simulink model "physbe"  (Simulink 9.0)
settings: Solver=ode45  StartTime=0.0  StopTime=20  FixedStep=1/1000  MaxStep=1/10  RelTol=1e-3  AbsTol=1e-6
PreLoadFcn:
  | pctrl2
values from neighbouring files (symbols this model uses):
  A = [  0.0   0.0   0.0  0.0  3.67   1.4   6.0   7.0  0.0  0.0 ]'*1000    [pctrl2.m]    (also in physbe_settings.mat = [0 0 0 0 3670 1400 6000 7000 0 0])
  C = [   75  5.33 75.00 1.01  4.25  1.21  34.0  11.1  250 32.5 ]'    [pctrl2.m]    (also in physbe_settings.mat = [75 7.519 80 1.25 4.25 1.21 34 11.1 250 30.3 2.57 5.33 ... ()
  Cl = [ 0.0000 0.04 0.08 0.12 0.16 0.20 0.24 0.28 0.32 0.36 0.4000 1.0000 ... (first row only)    [pctrl2.m]    (also in physbe_settings.mat = [0 0.00264 0.016 0.24 0.032 0.4 0.048 0.5 0.064 0.56 0.08 0.)
  Cr = [ 0.0000 0.04 0.08 0.12 0.16 0.20 0.24 0.28 0.32 0.36 0.4000 1.0000 ... (first row only)    [pctrl2.m]    (also in physbe_settings.mat = [0 0.00132 0.016 0.02 0.032 0.04 0.048 0.06 0.064 0.068 0.08)
  fd = fe    [pctrl2.m]    (also in physbe_settings.mat = [0 0 0 0 0 0 0 0 0 0])
  fe = [  0.0   0.0   0.0  0.0   0.0   0.0   0.0   0.0  0.0  0.0 ]'    [pctrl2.m]    (also in physbe_settings.mat = [0 0 0 0 0 0 0 0 0 0])
  h0 = [  0.0   0.0   0.0  0.0   0.0   0.0   0.0   0.0  0.0  0.0 ]'    [pctrl2.m]    (also in physbe_settings.mat = [0 0 0 0 0 0 0 0 0 0 0 0 ... (20 elements, 10x2)])
  K = 1    [pctrl2.m]    (also in physbe_settings.mat)
  Ri = [  3.0 187.5  27.5    0  5150  2580   670  2580  0.0  0.0 ]'*0.001    [pctrl2.m]    (also in physbe_settings.mat = [0.0128 0.1429 0.0588 0 5.15 2.58 0.67 2.58 0 0])
  Ro = [ 3e-3   0.0  6e-3    0    10     5  1.42     5  0.0  0.0 ]'    [pctrl2.m]    (also in physbe_settings.mat = [0.0111 0 0.0125 0 10 5 1.42 5 0 0])
  ta = 300    [pctrl2.m]    (also in physbe_settings.mat)
  V0 = [  150   120   150  100   280  80.0  2250   730  500  240 ]'    [pctrl2.m]    (also in physbe_settings.mat = [150 120 150 100 280 80 2250 730 500 240 2.57 120 ... (20 el)
  W = [  0.6   1.0   0.6  0.0  7.00   4.5  53.0  18.5  0.0  0.0 ]'*1000    [pctrl2.m]    (also in physbe_settings.mat = [600 1000 600 0 7000 4500 53000 18500 0 0])
libraries: simulink x2
CloseFcn:
  | close(findobj(allchild(0),'flat','name','PHYSBE Control Center'))
settings Model: Creator=anast  LastModifiedBy=anast  ExtModeTrigMode=oneshot  ExtModeArmWhenConnect=off
settings DataIOCC: Decimation=10  LimitDataPoints=on  SignalLoggingSaveFormat=ModelDataLogs
settings OptimizationCC: BlockReduction=off  BooleanDataType=off  LifeSpan=auto
settings DebuggingCC: ConsistencyChecking=warning  SaveWithParameterizedLinksMsg=none  SignalResolutionControl=TryResolveAllWithWarning  MultiTaskDSMMsg=warning  MultiTaskCondExecSysMsg=none  SFUnexpectedBacktrackingDiag=error  SFNoUnconditionalDefaultTransitionDiag=error  SFExecutionAtInitializationDiag=warning
settings HardwareCC: ProdBitPerPointer=64  ProdBitPerSizeT=64  ProdBitPerPtrDiffT=64  ProdLargestAtomicFloat=Float  ProdIntDivRoundTo=Zero  ProdEndianess=LittleEndian  ProdWordSize=64  ProdHWDeviceType=Intel->x86-64 (Windows64)  TargetUnknown=on
settings CodeAppCC: StateflowObjectComments=off
settings GRTTargetCC: CombineOutputUpdateFcns=off  GRTInterface=on
settings ConfigComp: CovMetricSettings=dwe  CovHtmlReporting=off  CovSaveCumulativeToWorkspaceVar=off  CovSaveSingleToWorkspaceVar=off  CovExternalEMLEnable=on

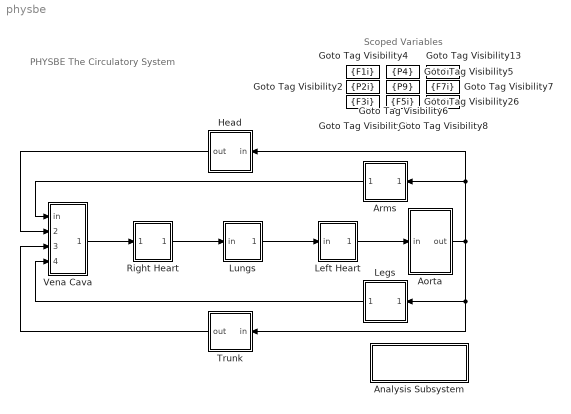
== system physbe ==
  note: Scoped Variables
  note: PHYSBE
      |  The Circulatory System
  Analysis Subsystem : Subsystem
      mask Display: disp('Analysis\nSubsystem')
  Aorta : Subsystem
      mask Display: disp('AORTA')
  Arms : Subsystem
      mask Display: disp('ARMS')
  Goto Tag Visibility13 : GotoTagVisibility  GotoTag=F6i
  Goto Tag Visibility2 : GotoTagVisibility  GotoTag=P2i
  Goto Tag Visibility26 : GotoTagVisibility  GotoTag=F5i
  Goto Tag Visibility3 : GotoTagVisibility  GotoTag=F3i
  Goto Tag Visibility4 : GotoTagVisibility  GotoTag=F1i
  Goto Tag Visibility5 : GotoTagVisibility  GotoTag=P4
  Goto Tag Visibility6 : GotoTagVisibility  GotoTag=P9
  Goto Tag Visibility7 : GotoTagVisibility  GotoTag=F7i
  Goto Tag Visibility8 : GotoTagVisibility  GotoTag=F8i
  Head : Subsystem
      mask Display: disp('HEAD')
  Left Heart : Subsystem
      mask Display: disp(' LEFT\n HEART')
  Legs : Subsystem
      mask Display: disp('LEGS')
  Lungs : Subsystem
      mask Display: disp('LUNGS')
  Right Heart : Subsystem
      mask Display: disp(' RIGHT\n HEART')
  Trunk : Subsystem
      mask Display: disp('TRUNK')
  Vena Cava : Subsystem
      mask Display: disp('VENA\nCAVA')
  wires:
  Arms/1(out1) -> Vena Cava/1(in)
  Head/1(out) -> Vena Cava/2(in1)
  Aorta/1(out) -> Legs/1(in1), Trunk/1(in), Arms/1(in1), Head/1(in)
  Lungs/1(out) -> Left Heart/1(in)
  Right Heart/1(out1) -> Lungs/1(in)
  Vena Cava/1(out) -> Right Heart/1(in1)
  Left Heart/1(out) -> Aorta/1(in)
  Legs/1(out1) -> Vena Cava/4(in3)
  Trunk/1(out) -> Vena Cava/3(in2)

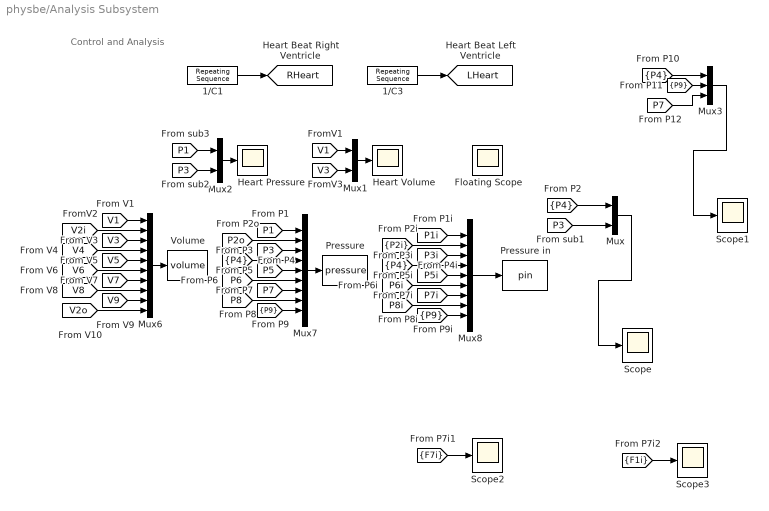
== system physbe/Analysis Subsystem ==
  note: Control
      | and
      |  Analysis
  1/C1 : simulink/Sources/Repeating Sequence  rep_seq_t=Cr(1,:)  rep_seq_y=Cr(2,:)
  1/C3 : simulink/Sources/Repeating Sequence  rep_seq_t=Cl(1,:)  rep_seq_y=Cl(2,:)
  Floating Scope : Scope
      settings: Floating=on
  Heart Pressure : Scope
  Heart Volume : Scope
  Mux : Mux  Inputs=2
  Mux1 : Mux  Inputs=2
  Mux2 : Mux  Inputs=2
  Mux3 : Mux  Inputs=3
  Mux6 : Mux  Inputs=10
  Mux7 : Mux  Inputs=9
  Mux8 : Mux  Inputs=9
  Pressure : ToWorkspace  VariableName=pressure  SampleTime=-1
      settings: Decimation=10
  Pressure in : ToWorkspace  VariableName=pin  SampleTime=-1
      settings: Decimation=10
  Scope{,1..3} (4 alike) : Scope
  Volume : ToWorkspace  VariableName=volume  SampleTime=-1
      settings: Decimation=10
  tag scope: LHeart=global, RHeart=global
  wires:
  Mux8/1 -> Pressure in/1
  [P7i] -> Mux8/7
  [P5i] -> Mux8/5
  [P3i] -> Mux8/3
  [P1i] -> Mux8/1
  [P9] -> Mux8/9
  [P7] -> Mux7/7
  [P3] -> Mux7/3
  [P5] -> Mux7/5
  [P9] -> Mux7/9
  Mux7/1 -> Pressure/1
  [P1] -> Mux7/1
  [V2o] -> Mux6/10
  [V2i] -> Mux6/2
  [V6] -> Mux6/6
  [V4] -> Mux6/4
  [V5] -> Mux6/5
  [V3] -> Mux6/3
  [V7] -> Mux6/7
  [V8] -> Mux6/8
  Mux6/1 -> Volume/1
  [V9] -> Mux6/9
  [V1] -> Mux6/1
  [P2o] -> Mux7/2
  [P6] -> Mux7/6
  [P8] -> Mux7/8
  [P4] -> Mux7/4
  [P8i] -> Mux8/8
  [P6i] -> Mux8/6
  [P4] -> Mux8/4
  [P2i] -> Mux8/2
  [P1] -> Mux2/1
  [V1] -> Mux1/1
  Mux1/1 -> Heart Volume/1
  [P3] -> Mux2/2
  Mux2/1 -> Heart Pressure/1
  [V3] -> Mux1/2
  1/C3/1 -> [LHeart]
  1/C1/1 -> [RHeart]
  [P3] -> Mux/2
  Mux/1 -> Scope/1
  [P4] -> Mux/1
  Mux3/1 -> Scope1/1
  [P4] -> Mux3/1
  [P9] -> Mux3/2
  [P7] -> Mux3/3
  [F7i] -> Scope2/1
  [F1i] -> Scope3/1

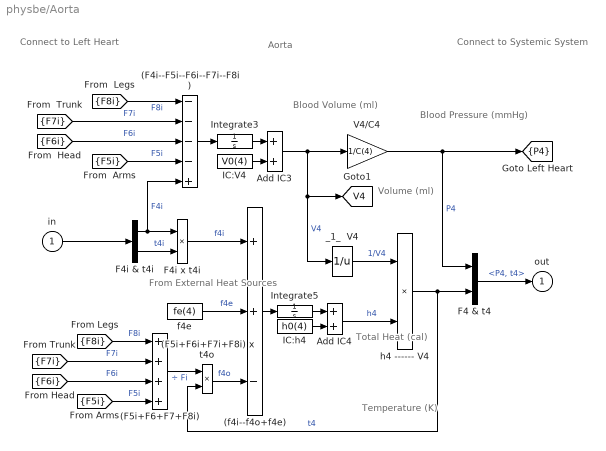
== system physbe/Aorta ==
  note: Temperature
      | (K)
  note: Volume
      | (ml)
  note: Connect to
      | Left Heart
  note: Connect to
      | Systemic System
  note: From External
      | Heat Sources
  note: Blood
      | Pressure
      | (mmHg)
  note: Total
      | Heat
      | (cal)
  note: Blood
      |  Volume
      | (ml)
  note: Aorta
  in : Inport
  (F4i--F5i--F6i--F7i--F8i) : Sum  Inputs=----+  SaturateOnIntegerOverflow=on  InputSameDT=on  OutDataTypeStr=Inherit: Same as first input
  (F5i+F6+F7+F8i) : Sum  Inputs=++++  SaturateOnIntegerOverflow=on  InputSameDT=on  OutDataTypeStr=Inherit: Same as first input
  (F5i+F6i+F7i+F8i) x t4o : Product  SaturateOnIntegerOverflow=on  RndMeth=Zero  InputSameDT=on  OutDataTypeStr=Inherit: Same as first input
  (f4i--f4o+f4e) : Sum  Inputs=++-  SaturateOnIntegerOverflow=on  InputSameDT=on  OutDataTypeStr=Inherit: Same as first input
  Add IC3 : Sum  SaturateOnIntegerOverflow=on  InputSameDT=on  OutDataTypeStr=Inherit: Same as first input
  Add IC4 : Sum  SaturateOnIntegerOverflow=on  InputSameDT=on  OutDataTypeStr=Inherit: Same as first input
  F4 & t4 : Mux  Inputs=2
  F4i & t4i : Demux  Outputs=2
  F4i x t4i : Product  SaturateOnIntegerOverflow=on  RndMeth=Zero  InputSameDT=on  OutDataTypeStr=Inherit: Same as first input
  IC:V4 : Constant  Value=V0(4)
  IC:h4 : Constant  Value=h0(4)
  Integrate3 : Integrator
  Integrate5 : Integrator
  V4/C4 : Gain  Gain=1/C(4)  SaturateOnIntegerOverflow=on  OutDataTypeStr=Inherit: Same as input  ParamDataTypeStr=Inherit: Same as input
  _1_  V4 : Math  Operator=reciprocal  SaturateOnIntegerOverflow=on
  f4e : Constant  Value=fe(4)
  h4 ------ V4 : Product  SaturateOnIntegerOverflow=on  RndMeth=Zero  InputSameDT=on  OutDataTypeStr=Inherit: Same as first input
  out : Outport
  tag scope: P4=scoped, V4=global
  wires:
  Integrate5/1 -> Add IC4/1
  IC:h4/1 -> Add IC4/2
  Integrate3/1 -> Add IC3/1
  IC:V4/1 -> Add IC3/2
  F4 & t4/1 -> out/1  "<P4, t4>"
  [F7i] -> (F4i--F5i--F6i--F7i--F8i)/2  "F7i"
  [F6i] -> (F4i--F5i--F6i--F7i--F8i)/3  "F6i"
  in/1 -> F4i & t4i/1
  [F7i] -> (F5i+F6+F7+F8i)/2  "F7i"
  [F6i] -> (F5i+F6+F7+F8i)/3  "F6i"
  [F8i] -> (F5i+F6+F7+F8i)/1  "F8i"
  [F5i] -> (F5i+F6+F7+F8i)/4  "F5i"
  (F5i+F6+F7+F8i)/1 -> (F5i+F6i+F7i+F8i) x t4o/1  "÷ Fi"
  F4i x t4i/1 -> (f4i--f4o+f4e)/1  "f4i"
  F4i & t4i/1 -> F4i x t4i/1, (F4i--F5i--F6i--F7i--F8i)/5  "F4i"
  F4i & t4i/2 -> F4i x t4i/2  "t4i"
  f4e/1 -> (f4i--f4o+f4e)/2  "f4e"
  [F8i] -> (F4i--F5i--F6i--F7i--F8i)/1  "F8i"
  [F5i] -> (F4i--F5i--F6i--F7i--F8i)/4  "F5i"
  V4/C4/1 -> [P4], F4 & t4/1  "P4"
  Add IC3/1 -> V4/C4/1, _1_  V4/1, [V4]  "V4"
  Add IC4/1 -> h4 ------ V4/2  "h4"
  _1_  V4/1 -> h4 ------ V4/1  "1/V4"
  h4 ------ V4/1 -> (F5i+F6i+F7i+F8i) x t4o/2, F4 & t4/2  "t4"
  (f4i--f4o+f4e)/1 -> Integrate5/1
  (F5i+F6i+F7i+F8i) x t4o/1 -> (f4i--f4o+f4e)/3  "f4o"
  (F4i--F5i--F6i--F7i--F8i)/1 -> Integrate3/1

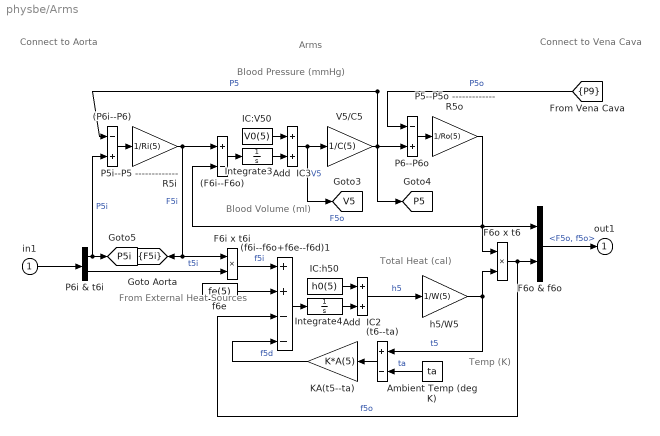
== system physbe/Arms ==
  note: From External
      | Heat Sources
  note: Blood Volume
      | (ml)
  note: Blood Pressure (mmHg)
  note: Total
      | Heat
      |  (cal)
  note: Temp
      | (K)
  note: Connect to
      | Vena Cava
  note: Arms
  note: Connect to
      | Aorta
  in1 : Inport
  (F6i--F6o) : Sum  Inputs=+-  SaturateOnIntegerOverflow=on  InputSameDT=on  OutDataTypeStr=Inherit: Same as first input
  (P6i--P6) : Sum  Inputs=-+  SaturateOnIntegerOverflow=on  InputSameDT=on  OutDataTypeStr=Inherit: Same as first input
  (f6i--f6o+f6e--f6d)1 : Sum  Inputs=++--  SaturateOnIntegerOverflow=on  InputSameDT=on  OutDataTypeStr=Inherit: Same as first input
  (t6--ta) : Sum  Inputs=+-  SaturateOnIntegerOverflow=on  InputSameDT=on  OutDataTypeStr=Inherit: Same as first input
  Add  IC2 : Sum  SaturateOnIntegerOverflow=on  InputSameDT=on  OutDataTypeStr=Inherit: Same as first input
  Add  IC3 : Sum  SaturateOnIntegerOverflow=on  InputSameDT=on  OutDataTypeStr=Inherit: Same as first input
  Ambient Temp (deg K) : Constant  Value=ta
  F6i x t6i : Product  SaturateOnIntegerOverflow=on  RndMeth=Zero  InputSameDT=on  OutDataTypeStr=Inherit: Same as first input
  F6o & f6o : Mux  Inputs=2
  F6o x t6 : Product  SaturateOnIntegerOverflow=on  RndMeth=Zero  InputSameDT=on  OutDataTypeStr=Inherit: Same as first input
  IC:V50 : Constant  Value=V0(5)
  IC:h50 : Constant  Value=h0(5)
  Integrate3 : Integrator
  Integrate4 : Integrator
  KA(t5--ta) : Gain  Gain=K*A(5)  SaturateOnIntegerOverflow=on  OutDataTypeStr=Inherit: Same as input  ParamDataTypeStr=Inherit: Same as input
  P5--P5o ------------- R5o : Gain  Gain=1/Ro(5)  SaturateOnIntegerOverflow=on  OutDataTypeStr=Inherit: Same as input  ParamDataTypeStr=Inherit: Same as input
  P5i--P5 ------------- R5i : Gain  Gain=1/Ri(5)  SaturateOnIntegerOverflow=on  OutDataTypeStr=Inherit: Same as input  ParamDataTypeStr=Inherit: Same as input
  P6--P6o : Sum  Inputs=-+  SaturateOnIntegerOverflow=on  InputSameDT=on  OutDataTypeStr=Inherit: Same as first input
  P6i & t6i : Demux  Outputs=2
  V5/C5 : Gain  Gain=1/C(5)  SaturateOnIntegerOverflow=on  OutDataTypeStr=Inherit: Same as input  ParamDataTypeStr=Inherit: Same as input
  f6e : Constant  Value=fe(5)
  h5/W5 : Gain  Gain=1/W(5)  SaturateOnIntegerOverflow=on  OutDataTypeStr=Inherit: Same as input  ParamDataTypeStr=Inherit: Same as input
  out1 : Outport
  tag scope: F5i=scoped, P5=global, P5i=global, V5=global
  wires:
  P6i & t6i/1 -> [P5i], (P6i--P6)/2  "P5i"
  h5/W5/1 -> (t6--ta)/1, F6o x t6/2  "t5"
  Ambient Temp (deg K)/1 -> (t6--ta)/2  "ta"
  (t6--ta)/1 -> KA(t5--ta)/1
  KA(t5--ta)/1 -> (f6i--f6o+f6e--f6d)1/4  "f5d"
  P5--P5o ------------- R5o/1 -> F6o x t6/1, F6o & f6o/1, (F6i--F6o)/2  "F5o"
  P6--P6o/1 -> P5--P5o ------------- R5o/1
  [P9] -> P6--P6o/1  "P5o"
  V5/C5/1 -> P6--P6o/2, (P6i--P6)/1, [P5]  "P5"
  Add  IC3/1 -> V5/C5/1, [V5]  "V5"
  Integrate3/1 -> Add  IC3/2
  IC:V50/1 -> Add  IC3/1
  F6o x t6/1 -> F6o & f6o/2, (f6i--f6o+f6e--f6d)1/3  "f5o"
  F6o & f6o/1 -> out1/1  "<F5o, f5o>"
  IC:h50/1 -> Add  IC2/1
  Integrate4/1 -> Add  IC2/2
  Add  IC2/1 -> h5/W5/1  "h5"
  f6e/1 -> (f6i--f6o+f6e--f6d)1/2
  F6i x t6i/1 -> (f6i--f6o+f6e--f6d)1/1  "f5i"
  (f6i--f6o+f6e--f6d)1/1 -> Integrate4/1
  P6i & t6i/2 -> F6i x t6i/2  "t5i"
  (P6i--P6)/1 -> P5i--P5 ------------- R5i/1
  P5i--P5 ------------- R5i/1 -> (F6i--F6o)/1, [F5i], F6i x t6i/1  "F5i"
  (F6i--F6o)/1 -> Integrate3/1
  in1/1 -> P6i & t6i/1

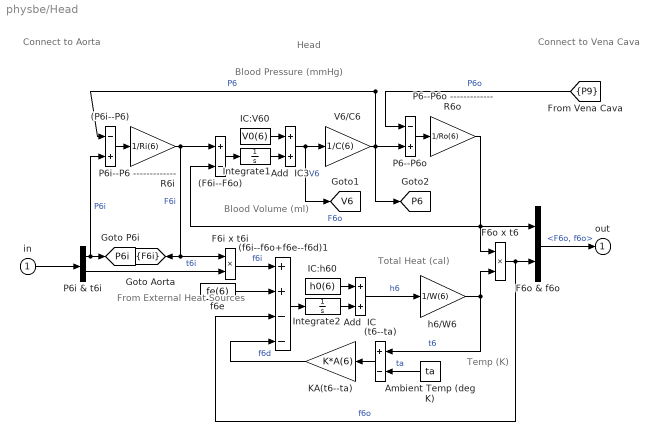
== system physbe/Head ==
  note: Connect to
      | Vena Cava
  note: From External
      | Heat Sources
  note: Head
  note: Blood Volume
      | (ml)
  note: Blood Pressure (mmHg)
  note: Total
      | Heat
      |  (cal)
  note: Temp
      | (K)
  note: Connect to
      | Aorta
  in : Inport
  (F6i--F6o) : Sum  Inputs=+-  SaturateOnIntegerOverflow=on  InputSameDT=on  OutDataTypeStr=Inherit: Same as first input
  (P6i--P6) : Sum  Inputs=-+  SaturateOnIntegerOverflow=on  InputSameDT=on  OutDataTypeStr=Inherit: Same as first input
  (f6i--f6o+f6e--f6d)1 : Sum  Inputs=++--  SaturateOnIntegerOverflow=on  InputSameDT=on  OutDataTypeStr=Inherit: Same as first input
  (t6--ta) : Sum  Inputs=+-  SaturateOnIntegerOverflow=on  InputSameDT=on  OutDataTypeStr=Inherit: Same as first input
  Add  IC : Sum  SaturateOnIntegerOverflow=on  InputSameDT=on  OutDataTypeStr=Inherit: Same as first input
  Add  IC3 : Sum  SaturateOnIntegerOverflow=on  InputSameDT=on  OutDataTypeStr=Inherit: Same as first input
  Ambient Temp (deg K) : Constant  Value=ta
  F6i x t6i : Product  SaturateOnIntegerOverflow=on  RndMeth=Zero  InputSameDT=on  OutDataTypeStr=Inherit: Same as first input
  F6o & f6o : Mux  Inputs=2
  F6o x t6 : Product  SaturateOnIntegerOverflow=on  RndMeth=Zero  InputSameDT=on  OutDataTypeStr=Inherit: Same as first input
  IC:V60 : Constant  Value=V0(6)
  IC:h60 : Constant  Value=h0(6)
  Integrate1 : Integrator
  Integrate2 : Integrator
  KA(t6--ta) : Gain  Gain=K*A(6)  SaturateOnIntegerOverflow=on  OutDataTypeStr=Inherit: Same as input  ParamDataTypeStr=Inherit: Same as input
  P6--P6o : Sum  Inputs=-+  SaturateOnIntegerOverflow=on  InputSameDT=on  OutDataTypeStr=Inherit: Same as first input
  P6--P6o ------------- R6o : Gain  Gain=1/Ro(6)  SaturateOnIntegerOverflow=on  OutDataTypeStr=Inherit: Same as input  ParamDataTypeStr=Inherit: Same as input
  P6i & t6i : Demux  Outputs=2
  P6i--P6 ------------- R6i : Gain  Gain=1/Ri(6)  SaturateOnIntegerOverflow=on  OutDataTypeStr=Inherit: Same as input  ParamDataTypeStr=Inherit: Same as input
  V6/C6 : Gain  Gain=1/C(6)  SaturateOnIntegerOverflow=on  OutDataTypeStr=Inherit: Same as input  ParamDataTypeStr=Inherit: Same as input
  f6e : Constant  Value=fe(6)
  h6/W6 : Gain  Gain=1/W(6)  SaturateOnIntegerOverflow=on  OutDataTypeStr=Inherit: Same as input  ParamDataTypeStr=Inherit: Same as input
  out : Outport
  tag scope: F6i=scoped, P6=global, P6i=global, V6=global
  wires:
  P6i & t6i/1 -> [P6i], (P6i--P6)/2  "P6i"
  h6/W6/1 -> (t6--ta)/1, F6o x t6/2  "t6"
  Ambient Temp (deg K)/1 -> (t6--ta)/2  "ta"
  (t6--ta)/1 -> KA(t6--ta)/1
  KA(t6--ta)/1 -> (f6i--f6o+f6e--f6d)1/4  "f6d"
  P6--P6o ------------- R6o/1 -> F6o x t6/1, F6o & f6o/1, (F6i--F6o)/2  "F6o"
  P6--P6o/1 -> P6--P6o ------------- R6o/1
  [P9] -> P6--P6o/1  "P6o"
  V6/C6/1 -> P6--P6o/2, (P6i--P6)/1, [P6]  "P6"
  Add  IC3/1 -> V6/C6/1, [V6]  "V6"
  F6o x t6/1 -> F6o & f6o/2, (f6i--f6o+f6e--f6d)1/3  "f6o"
  F6o & f6o/1 -> out/1  "<F6o, f6o>"
  IC:h60/1 -> Add  IC/1
  Integrate2/1 -> Add  IC/2
  Add  IC/1 -> h6/W6/1  "h6"
  f6e/1 -> (f6i--f6o+f6e--f6d)1/2
  F6i x t6i/1 -> (f6i--f6o+f6e--f6d)1/1  "f6i"
  (f6i--f6o+f6e--f6d)1/1 -> Integrate2/1
  P6i & t6i/2 -> F6i x t6i/2  "t6i"
  in/1 -> P6i & t6i/1
  (P6i--P6)/1 -> P6i--P6 ------------- R6i/1
  P6i--P6 ------------- R6i/1 -> (F6i--F6o)/1, [F6i], F6i x t6i/1  "F6i"
  Integrate1/1 -> Add  IC3/2
  (F6i--F6o)/1 -> Integrate1/1
  IC:V60/1 -> Add  IC3/1

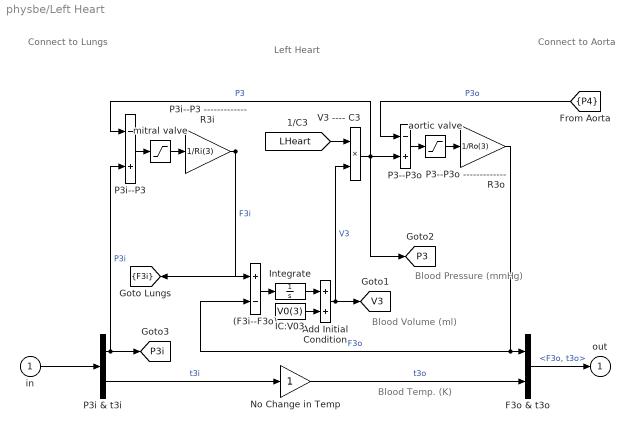
== system physbe/Left Heart ==
  note: Left Heart
  note: Connect to
      | Lungs
  note: Blood Volume (ml)
  note: Blood Pressure
      | (mmHg)
  note: Connect to
      | Aorta
  note: Blood Temp. (K)
  in : Inport
  (F3i--F3o) : Sum  Inputs=+-  SaturateOnIntegerOverflow=on  InputSameDT=on  OutDataTypeStr=Inherit: Same as first input
  Add Initial Condition : Sum  SaturateOnIntegerOverflow=on  InputSameDT=on  OutDataTypeStr=Inherit: Same as first input
  F3o & t3o : Mux  Inputs=2
  IC:V03 : Constant  Value=V0(3)
  Integrate : Integrator
  No Change in Temp : Gain  SaturateOnIntegerOverflow=on  OutDataTypeStr=Inherit: Same as input  ParamDataTypeStr=Inherit: Same as input
  P3--P3o : Sum  Inputs=-+  SaturateOnIntegerOverflow=on  InputSameDT=on  OutDataTypeStr=Inherit: Same as first input
  P3--P3o ------------- R3o : Gain  Gain=1/Ro(3)  SaturateOnIntegerOverflow=on  OutDataTypeStr=Inherit: Same as input  ParamDataTypeStr=Inherit: Same as input
  P3i & t3i : Demux  Outputs=2
  P3i--P3 : Sum  Inputs=-+  SaturateOnIntegerOverflow=on  InputSameDT=on  OutDataTypeStr=Inherit: Same as first input
  P3i--P3 ------------- R3i : Gain  Gain=1/Ri(3)  SaturateOnIntegerOverflow=on  OutDataTypeStr=Inherit: Same as input  ParamDataTypeStr=Inherit: Same as input
  V3 ---- C3 : Product  SaturateOnIntegerOverflow=on  RndMeth=Zero  InputSameDT=on  OutDataTypeStr=Inherit: Same as first input
  aortic valve : Saturate  UpperLimit=inf  LowerLimit=0
  mitral valve : Saturate  UpperLimit=inf  LowerLimit=0
  out : Outport
  tag scope: F3i=scoped, P3=global, P3i=global, V3=global
  wires:
  P3i & t3i/1 -> [P3i], P3i--P3/2  "P3i"
  P3i--P3 ------------- R3i/1 -> [F3i], (F3i--F3o)/1  "F3i"
  P3i--P3/1 -> mitral valve/1
  mitral valve/1 -> P3i--P3 ------------- R3i/1
  in/1 -> P3i & t3i/1
  Add Initial Condition/1 -> [V3], V3 ---- C3/2  "V3"
  P3i & t3i/2 -> No Change in Temp/1  "t3i"
  (F3i--F3o)/1 -> Integrate/1
  Integrate/1 -> Add Initial Condition/1
  IC:V03/1 -> Add Initial Condition/2
  [LHeart] -> V3 ---- C3/1
  P3--P3o/1 -> aortic valve/1
  aortic valve/1 -> P3--P3o ------------- R3o/1
  V3 ---- C3/1 -> P3i--P3/1, [P3], P3--P3o/2  "P3"
  No Change in Temp/1 -> F3o & t3o/2  "t3o"
  F3o & t3o/1 -> out/1  "<F3o, t3o>"
  P3--P3o ------------- R3o/1 -> F3o & t3o/1, (F3i--F3o)/2  "F3o"
  [P4] -> P3--P3o/1  "P3o"

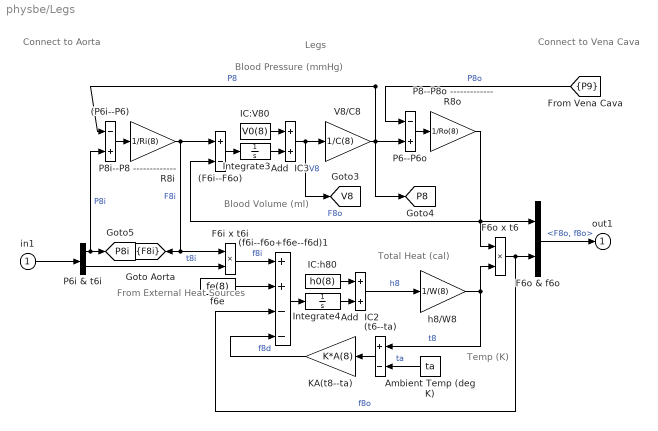
== system physbe/Legs ==
  note: From External
      | Heat Sources
  note: Blood Volume
      | (ml)
  note: Blood Pressure (mmHg)
  note: Total
      | Heat
      |  (cal)
  note: Temp
      | (K)
  note: Connect to
      | Vena Cava
  note: Legs
  note: Connect to
      | Aorta
  in1 : Inport
  (F6i--F6o) : Sum  Inputs=+-  SaturateOnIntegerOverflow=on  InputSameDT=on  OutDataTypeStr=Inherit: Same as first input
  (P6i--P6) : Sum  Inputs=-+  SaturateOnIntegerOverflow=on  InputSameDT=on  OutDataTypeStr=Inherit: Same as first input
  (f6i--f6o+f6e--f6d)1 : Sum  Inputs=++--  SaturateOnIntegerOverflow=on  InputSameDT=on  OutDataTypeStr=Inherit: Same as first input
  (t6--ta) : Sum  Inputs=+-  SaturateOnIntegerOverflow=on  InputSameDT=on  OutDataTypeStr=Inherit: Same as first input
  Add  IC2 : Sum  SaturateOnIntegerOverflow=on  InputSameDT=on  OutDataTypeStr=Inherit: Same as first input
  Add  IC3 : Sum  SaturateOnIntegerOverflow=on  InputSameDT=on  OutDataTypeStr=Inherit: Same as first input
  Ambient Temp (deg K) : Constant  Value=ta
  F6i x t6i : Product  SaturateOnIntegerOverflow=on  RndMeth=Zero  InputSameDT=on  OutDataTypeStr=Inherit: Same as first input
  F6o & f6o : Mux  Inputs=2
  F6o x t6 : Product  SaturateOnIntegerOverflow=on  RndMeth=Zero  InputSameDT=on  OutDataTypeStr=Inherit: Same as first input
  IC:V80 : Constant  Value=V0(8)
  IC:h80 : Constant  Value=h0(8)
  Integrate3 : Integrator
  Integrate4 : Integrator
  KA(t8--ta) : Gain  Gain=K*A(8)  SaturateOnIntegerOverflow=on  OutDataTypeStr=Inherit: Same as input  ParamDataTypeStr=Inherit: Same as input
  P6--P6o : Sum  Inputs=-+  SaturateOnIntegerOverflow=on  InputSameDT=on  OutDataTypeStr=Inherit: Same as first input
  P6i & t6i : Demux  Outputs=2
  P8--P8o ------------- R8o : Gain  Gain=1/Ro(8)  SaturateOnIntegerOverflow=on  OutDataTypeStr=Inherit: Same as input  ParamDataTypeStr=Inherit: Same as input
  P8i--P8 ------------- R8i : Gain  Gain=1/Ri(8)  SaturateOnIntegerOverflow=on  OutDataTypeStr=Inherit: Same as input  ParamDataTypeStr=Inherit: Same as input
  V8/C8 : Gain  Gain=1/C(8)  SaturateOnIntegerOverflow=on  OutDataTypeStr=Inherit: Same as input  ParamDataTypeStr=Inherit: Same as input
  f6e : Constant  Value=fe(8)
  h8/W8 : Gain  Gain=1/W(8)  SaturateOnIntegerOverflow=on  OutDataTypeStr=Inherit: Same as input  ParamDataTypeStr=Inherit: Same as input
  out1 : Outport
  tag scope: F8i=scoped, P8=global, P8i=global, V8=global
  wires:
  P6i & t6i/1 -> [P8i], (P6i--P6)/2  "P8i"
  h8/W8/1 -> (t6--ta)/1, F6o x t6/2  "t8"
  Ambient Temp (deg K)/1 -> (t6--ta)/2  "ta"
  (t6--ta)/1 -> KA(t8--ta)/1
  KA(t8--ta)/1 -> (f6i--f6o+f6e--f6d)1/4  "f8d"
  P8--P8o ------------- R8o/1 -> F6o x t6/1, F6o & f6o/1, (F6i--F6o)/2  "F8o"
  P6--P6o/1 -> P8--P8o ------------- R8o/1
  [P9] -> P6--P6o/1  "P8o"
  V8/C8/1 -> P6--P6o/2, (P6i--P6)/1, [P8]  "P8"
  Add  IC3/1 -> V8/C8/1, [V8]  "V8"
  Integrate3/1 -> Add  IC3/2
  IC:V80/1 -> Add  IC3/1
  F6o x t6/1 -> F6o & f6o/2, (f6i--f6o+f6e--f6d)1/3  "f8o"
  F6o & f6o/1 -> out1/1  "<F8o, f8o>"
  IC:h80/1 -> Add  IC2/1
  Integrate4/1 -> Add  IC2/2
  Add  IC2/1 -> h8/W8/1  "h8"
  f6e/1 -> (f6i--f6o+f6e--f6d)1/2
  F6i x t6i/1 -> (f6i--f6o+f6e--f6d)1/1  "f8i"
  (f6i--f6o+f6e--f6d)1/1 -> Integrate4/1
  P6i & t6i/2 -> F6i x t6i/2  "t8i"
  (P6i--P6)/1 -> P8i--P8 ------------- R8i/1
  P8i--P8 ------------- R8i/1 -> (F6i--F6o)/1, [F8i], F6i x t6i/1  "F8i"
  (F6i--F6o)/1 -> Integrate3/1
  in1/1 -> P6i & t6i/1

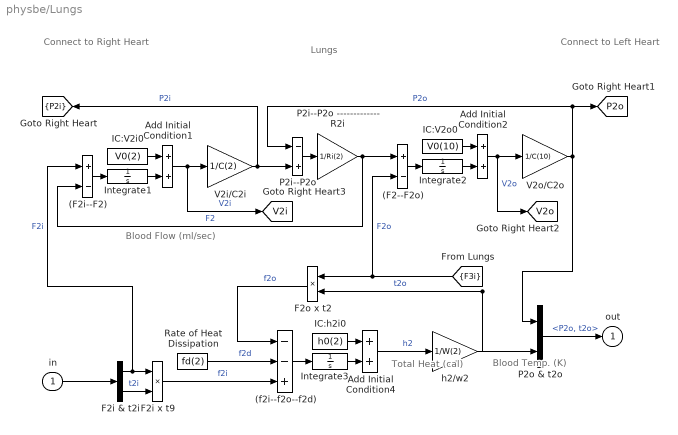
== system physbe/Lungs ==
  note: Connect to
      | Right Heart
  note: Connect to
      | Left Heart
  note: Blood
      | Temp.
      | (K)
  note: Total
      | Heat
      | (cal)
  note: Blood Flow (ml/sec)
  note: Lungs
  in : Inport
  (F2--F2o) : Sum  Inputs=+-  SaturateOnIntegerOverflow=on  InputSameDT=on  OutDataTypeStr=Inherit: Same as first input
  (F2i--F2) : Sum  Inputs=+-  SaturateOnIntegerOverflow=on  InputSameDT=on  OutDataTypeStr=Inherit: Same as first input
  (f2i--f2o--f2d) : Sum  Inputs=--+  SaturateOnIntegerOverflow=on  InputSameDT=on  OutDataTypeStr=Inherit: Same as first input
  Add Initial Condition1 : Sum  SaturateOnIntegerOverflow=on  InputSameDT=on  OutDataTypeStr=Inherit: Same as first input
  Add Initial Condition2 : Sum  SaturateOnIntegerOverflow=on  InputSameDT=on  OutDataTypeStr=Inherit: Same as first input
  Add Initial Condition4 : Sum  SaturateOnIntegerOverflow=on  InputSameDT=on  OutDataTypeStr=Inherit: Same as first input
  F2i & t2i : Demux  Outputs=2
  F2i x t9 : Product  SaturateOnIntegerOverflow=on  RndMeth=Zero  InputSameDT=on  OutDataTypeStr=Inherit: Same as first input
  F2o x t2 : Product  SaturateOnIntegerOverflow=on  RndMeth=Zero  InputSameDT=on  OutDataTypeStr=Inherit: Same as first input
  IC:V2i0 : Constant  Value=V0(2)
  IC:V2o0 : Constant  Value=V0(10)
  IC:h2i0 : Constant  Value=h0(2)
  Integrate1 : Integrator
  Integrate2 : Integrator
  Integrate3 : Integrator
  P2i--P2o : Sum  Inputs=-+  SaturateOnIntegerOverflow=on  InputSameDT=on  OutDataTypeStr=Inherit: Same as first input
  P2i--P2o ------------- R2i : Gain  Gain=1/Ri(2)  SaturateOnIntegerOverflow=on  OutDataTypeStr=Inherit: Same as input  ParamDataTypeStr=Inherit: Same as input
  P2o & t2o : Mux  Inputs=2
  Rate of Heat Dissipation : Constant  Value=fd(2)
  V2i/C2i : Gain  Gain=1/C(2)  SaturateOnIntegerOverflow=on  OutDataTypeStr=Inherit: Same as input  ParamDataTypeStr=Inherit: Same as input
  V2o/C2o : Gain  Gain=1/C(10)  SaturateOnIntegerOverflow=on  OutDataTypeStr=Inherit: Same as input  ParamDataTypeStr=Inherit: Same as input
  h2/w2 : Gain  Gain=1/W(2)  SaturateOnIntegerOverflow=on  OutDataTypeStr=Inherit: Same as input  ParamDataTypeStr=Inherit: Same as input
  out : Outport
  tag scope: P2i=scoped, P2o=global, V2i=global, V2o=global
  wires:
  Add Initial Condition1/1 -> [V2i], V2i/C2i/1  "V2i"
  Add Initial Condition2/1 -> [V2o], V2o/C2o/1  "V2o"
  (F2i--F2)/1 -> Integrate1/1
  IC:V2i0/1 -> Add Initial Condition1/1
  Integrate1/1 -> Add Initial Condition1/2
  P2o & t2o/1 -> out/1  "<P2o, t2o>"
  h2/w2/1 -> P2o & t2o/2, F2o x t2/2  "t2o"
  [F3i] -> F2o x t2/1, (F2--F2o)/2  "F2o"
  Integrate3/1 -> Add Initial Condition4/2
  (f2i--f2o--f2d)/1 -> Integrate3/1
  Add Initial Condition4/1 -> h2/w2/1  "h2"
  F2i x t9/1 -> (f2i--f2o--f2d)/3  "f2i"
  Rate of Heat Dissipation/1 -> (f2i--f2o--f2d)/2  "f2d"
  IC:h2i0/1 -> Add Initial Condition4/1
  F2o x t2/1 -> (f2i--f2o--f2d)/1  "f2o"
  P2i--P2o/1 -> P2i--P2o ------------- R2i/1
  P2i--P2o ------------- R2i/1 -> (F2--F2o)/1, (F2i--F2)/2  "F2"
  V2i/C2i/1 -> [P2i], P2i--P2o/2  "P2i"
  (F2--F2o)/1 -> Integrate2/1
  IC:V2o0/1 -> Add Initial Condition2/1
  Integrate2/1 -> Add Initial Condition2/2
  V2o/C2o/1 -> [P2o], P2i--P2o/1, P2o & t2o/1  "P2o"
  in/1 -> F2i & t2i/1
  F2i & t2i/1 -> F2i x t9/1, (F2i--F2)/1  "F2i"
  F2i & t2i/2 -> F2i x t9/2  "t2i"

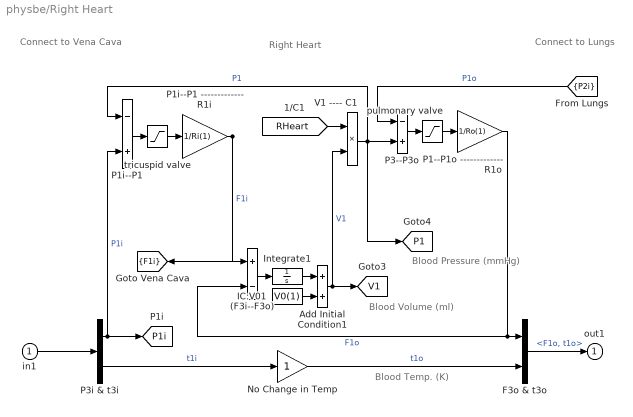
== system physbe/Right Heart ==
  note: Blood Volume (ml)
  note: Blood Pressure
      | (mmHg)
  note: Blood Temp. (K)
  note: Connect to
      | Lungs
  note: Connect to
      | Vena Cava
  note: Right Heart
  in1 : Inport
  (F3i--F3o) : Sum  Inputs=+-  SaturateOnIntegerOverflow=on  InputSameDT=on  OutDataTypeStr=Inherit: Same as first input
  Add Initial Condition1 : Sum  SaturateOnIntegerOverflow=on  InputSameDT=on  OutDataTypeStr=Inherit: Same as first input
  F3o & t3o : Mux  Inputs=2
  IC:V01 : Constant  Value=V0(1)
  Integrate1 : Integrator
  No Change in Temp : Gain  SaturateOnIntegerOverflow=on  OutDataTypeStr=Inherit: Same as input  ParamDataTypeStr=Inherit: Same as input
  P1--P1o ------------- R1o : Gain  Gain=1/Ro(1)  SaturateOnIntegerOverflow=on  OutDataTypeStr=Inherit: Same as input  ParamDataTypeStr=Inherit: Same as input
  P1i--P1 : Sum  Inputs=-+  SaturateOnIntegerOverflow=on  InputSameDT=on  OutDataTypeStr=Inherit: Same as first input
  P1i--P1 ------------- R1i : Gain  Gain=1/Ri(1)  SaturateOnIntegerOverflow=on  OutDataTypeStr=Inherit: Same as input  ParamDataTypeStr=Inherit: Same as input
  P3--P3o : Sum  Inputs=-+  SaturateOnIntegerOverflow=on  InputSameDT=on  OutDataTypeStr=Inherit: Same as first input
  P3i & t3i : Demux  Outputs=2
  V1 ---- C1 : Product  SaturateOnIntegerOverflow=on  RndMeth=Zero  InputSameDT=on  OutDataTypeStr=Inherit: Same as first input
  pulmonary valve : Saturate  UpperLimit=inf  LowerLimit=0
  tricuspid valve : Saturate  UpperLimit=inf  LowerLimit=0
  out1 : Outport
  tag scope: F1i=scoped, P1=global, P1i=global, V1=global
  wires:
  P3i & t3i/1 -> [P1i], P1i--P1/2  "P1i"
  P1i--P1 ------------- R1i/1 -> [F1i], (F3i--F3o)/1  "F1i"
  P1i--P1/1 -> tricuspid valve/1
  tricuspid valve/1 -> P1i--P1 ------------- R1i/1
  in1/1 -> P3i & t3i/1
  Add Initial Condition1/1 -> [V1], V1 ---- C1/2  "V1"
  P3i & t3i/2 -> No Change in Temp/1  "t1i"
  (F3i--F3o)/1 -> Integrate1/1
  Integrate1/1 -> Add Initial Condition1/1
  IC:V01/1 -> Add Initial Condition1/2
  [RHeart] -> V1 ---- C1/1
  P3--P3o/1 -> pulmonary valve/1
  pulmonary valve/1 -> P1--P1o ------------- R1o/1
  V1 ---- C1/1 -> P1i--P1/1, [P1], P3--P3o/2  "P1"
  No Change in Temp/1 -> F3o & t3o/2  "t1o"
  F3o & t3o/1 -> out1/1  "<F1o, t1o>"
  P1--P1o ------------- R1o/1 -> F3o & t3o/1, (F3i--F3o)/2  "F1o"
  [P2i] -> P3--P3o/1  "P1o"

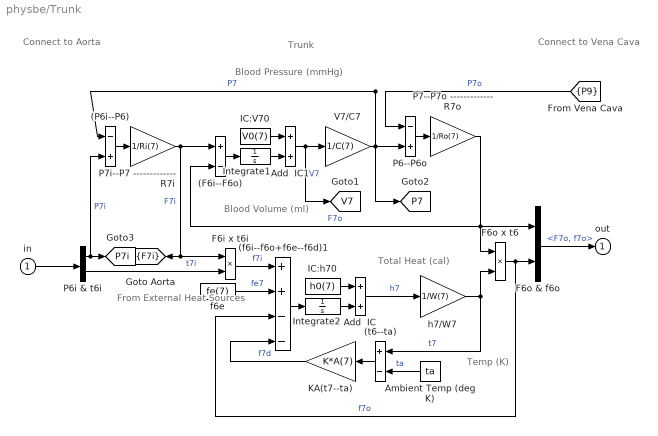
== system physbe/Trunk ==
  note: From External
      | Heat Sources
  note: Blood Volume
      | (ml)
  note: Blood Pressure (mmHg)
  note: Total
      | Heat
      |  (cal)
  note: Temp
      | (K)
  note: Connect to
      | Vena Cava
  note: Trunk
  note: Connect to
      | Aorta
  in : Inport
  (F6i--F6o) : Sum  Inputs=+-  SaturateOnIntegerOverflow=on  InputSameDT=on  OutDataTypeStr=Inherit: Same as first input
  (P6i--P6) : Sum  Inputs=-+  SaturateOnIntegerOverflow=on  InputSameDT=on  OutDataTypeStr=Inherit: Same as first input
  (f6i--f6o+f6e--f6d)1 : Sum  Inputs=++--  SaturateOnIntegerOverflow=on  InputSameDT=on  OutDataTypeStr=Inherit: Same as first input
  (t6--ta) : Sum  Inputs=+-  SaturateOnIntegerOverflow=on  InputSameDT=on  OutDataTypeStr=Inherit: Same as first input
  Add  IC : Sum  SaturateOnIntegerOverflow=on  InputSameDT=on  OutDataTypeStr=Inherit: Same as first input
  Add  IC1 : Sum  SaturateOnIntegerOverflow=on  InputSameDT=on  OutDataTypeStr=Inherit: Same as first input
  Ambient Temp (deg K) : Constant  Value=ta
  F6i x t6i : Product  SaturateOnIntegerOverflow=on  RndMeth=Zero  InputSameDT=on  OutDataTypeStr=Inherit: Same as first input
  F6o & f6o : Mux  Inputs=2
  F6o x t6 : Product  SaturateOnIntegerOverflow=on  RndMeth=Zero  InputSameDT=on  OutDataTypeStr=Inherit: Same as first input
  IC:V70 : Constant  Value=V0(7)
  IC:h70 : Constant  Value=h0(7)
  Integrate1 : Integrator
  Integrate2 : Integrator
  KA(t7--ta) : Gain  Gain=K*A(7)  SaturateOnIntegerOverflow=on  OutDataTypeStr=Inherit: Same as input  ParamDataTypeStr=Inherit: Same as input
  P6--P6o : Sum  Inputs=-+  SaturateOnIntegerOverflow=on  InputSameDT=on  OutDataTypeStr=Inherit: Same as first input
  P6i & t6i : Demux  Outputs=2
  P7--P7o ------------- R7o : Gain  Gain=1/Ro(7)  SaturateOnIntegerOverflow=on  OutDataTypeStr=Inherit: Same as input  ParamDataTypeStr=Inherit: Same as input
  P7i--P7 ------------- R7i : Gain  Gain=1/Ri(7)  SaturateOnIntegerOverflow=on  OutDataTypeStr=Inherit: Same as input  ParamDataTypeStr=Inherit: Same as input
  V7/C7 : Gain  Gain=1/C(7)  SaturateOnIntegerOverflow=on  OutDataTypeStr=Inherit: Same as input  ParamDataTypeStr=Inherit: Same as input
  f6e : Constant  Value=fe(7)
  h7/W7 : Gain  Gain=1/W(7)  SaturateOnIntegerOverflow=on  OutDataTypeStr=Inherit: Same as input  ParamDataTypeStr=Inherit: Same as input
  out : Outport
  tag scope: F7i=scoped, P7=global, P7i=global, V7=global
  wires:
  P6i & t6i/1 -> [P7i], (P6i--P6)/2  "P7i"
  h7/W7/1 -> (t6--ta)/1, F6o x t6/2  "t7"
  Ambient Temp (deg K)/1 -> (t6--ta)/2  "ta"
  (t6--ta)/1 -> KA(t7--ta)/1
  KA(t7--ta)/1 -> (f6i--f6o+f6e--f6d)1/4  "f7d"
  P7--P7o ------------- R7o/1 -> F6o x t6/1, F6o & f6o/1, (F6i--F6o)/2  "F7o"
  P6--P6o/1 -> P7--P7o ------------- R7o/1
  [P9] -> P6--P6o/1  "P7o"
  V7/C7/1 -> P6--P6o/2, (P6i--P6)/1, [P7]  "P7"
  Add  IC1/1 -> V7/C7/1, [V7]  "V7"
  Integrate1/1 -> Add  IC1/2
  IC:V70/1 -> Add  IC1/1
  F6o x t6/1 -> F6o & f6o/2, (f6i--f6o+f6e--f6d)1/3  "f7o"
  F6o & f6o/1 -> out/1  "<F7o, f7o>"
  IC:h70/1 -> Add  IC/1
  Integrate2/1 -> Add  IC/2
  Add  IC/1 -> h7/W7/1  "h7"
  f6e/1 -> (f6i--f6o+f6e--f6d)1/2  "fe7"
  F6i x t6i/1 -> (f6i--f6o+f6e--f6d)1/1  "f7i"
  (f6i--f6o+f6e--f6d)1/1 -> Integrate2/1
  P6i & t6i/2 -> F6i x t6i/2  "t7i"
  (P6i--P6)/1 -> P7i--P7 ------------- R7i/1
  P7i--P7 ------------- R7i/1 -> (F6i--F6o)/1, [F7i], F6i x t6i/1  "F7i"
  (F6i--F6o)/1 -> Integrate1/1
  in/1 -> P6i & t6i/1

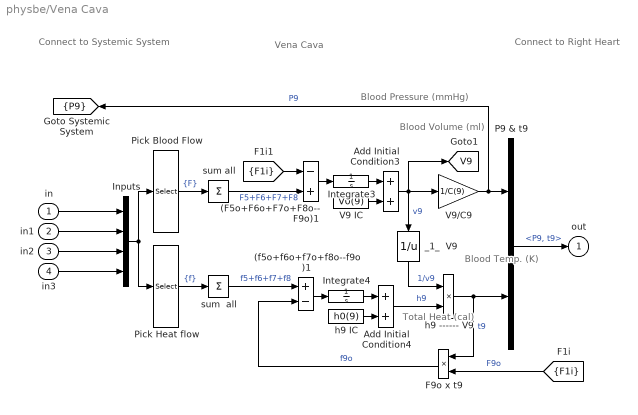
== system physbe/Vena Cava ==
  note: Total
      | Heat
      | (cal)
  note: Vena Cava
  note: Blood Pressure (mmHg)
  note: Blood
      | Temp.
      | (K)
  note: Blood
      |  Volume
      | (ml)
  note: Connect to
      | Right Heart
  note: Connect to
      | Systemic System
  in : Inport
  in1 : Inport  Port=2
  in2 : Inport  Port=3
  in3 : Inport  Port=4
  (F5o+F6o+F7o+F8o--F9o)1 : Sum  Inputs=-+  SaturateOnIntegerOverflow=on  InputSameDT=on  OutDataTypeStr=Inherit: Same as first input
  (f5o+f6o+f7o+f8o--f9o)1 : Sum  Inputs=+-  SaturateOnIntegerOverflow=on  InputSameDT=on  OutDataTypeStr=Inherit: Same as first input
  Add Initial Condition3 : Sum  SaturateOnIntegerOverflow=on  InputSameDT=on  OutDataTypeStr=Inherit: Same as first input
  Add Initial Condition4 : Sum  SaturateOnIntegerOverflow=on  InputSameDT=on  OutDataTypeStr=Inherit: Same as first input
  F9o x t9 : Product  SaturateOnIntegerOverflow=on  RndMeth=Zero  InputSameDT=on  OutDataTypeStr=Inherit: Same as first input
  Inputs : Mux
  Integrate3 : Integrator
  Integrate4 : Integrator
  P9 & t9 : Mux  Inputs=2
  Pick Blood Flow : Selector  InputPortWidth=8  IndexOptions=Index vector (dialog)  Indices=[1,3,5,7]  OutputSizes=1
  Pick Heat flow : Selector  InputPortWidth=8  IndexOptions=Index vector (dialog)  Indices=[2,4,6,8]  OutputSizes=1
  V9 IC : Constant  Value=V0(9)
  V9/C9 : Gain  Gain=1/C(9)  SaturateOnIntegerOverflow=on  OutDataTypeStr=Inherit: Same as input  ParamDataTypeStr=Inherit: Same as input
  _1_  V9 : Math  Operator=reciprocal  SaturateOnIntegerOverflow=on
  h9 ------ V9 : Product  SaturateOnIntegerOverflow=on  RndMeth=Zero  InputSameDT=on  OutDataTypeStr=Inherit: Same as first input
  h9 IC : Constant  Value=h0(9)
  sum  all : Sum  Inputs=1  SaturateOnIntegerOverflow=on  InputSameDT=on  OutDataTypeStr=Inherit: Same as first input
  sum all : Sum  Inputs=1  SaturateOnIntegerOverflow=on  InputSameDT=on  OutDataTypeStr=Inherit: Same as first input
  out : Outport
  tag scope: P9=scoped, V9=global
  wires:
  Add Initial Condition3/1 -> V9/C9/1, _1_  V9/1, [V9]  "v9"
  Inputs/1 -> Pick Heat flow/1, Pick Blood Flow/1
  [F1i] -> F9o x t9/2  "F9o"
  [F1i] -> (F5o+F6o+F7o+F8o--F9o)1/1
  sum all/1 -> (F5o+F6o+F7o+F8o--F9o)1/2  "F5+F6+F7+F8"
  Pick Blood Flow/1 -> sum all/1  "{F}"
  sum  all/1 -> (f5o+f6o+f7o+f8o--f9o)1/1  "f5+f6+f7+f8"
  Pick Heat flow/1 -> sum  all/1  "{f}"
  h9 ------ V9/1 -> F9o x t9/1, P9 & t9/2  "t9"
  (f5o+f6o+f7o+f8o--f9o)1/1 -> Integrate4/1
  in3/1 -> Inputs/4
  in2/1 -> Inputs/3
  in1/1 -> Inputs/2
  in/1 -> Inputs/1
  (F5o+F6o+F7o+F8o--F9o)1/1 -> Integrate3/1
  P9 & t9/1 -> out/1  "<P9, t9>"
  V9/C9/1 -> P9 & t9/1, [P9]  "P9"
  Integrate4/1 -> Add Initial Condition4/1
  h9 IC/1 -> Add Initial Condition4/2
  Integrate3/1 -> Add Initial Condition3/1
  V9 IC/1 -> Add Initial Condition3/2
  Add Initial Condition4/1 -> h9 ------ V9/2  "h9"
  _1_  V9/1 -> h9 ------ V9/1  "1/v9"
  F9o x t9/1 -> (f5o+f6o+f7o+f8o--f9o)1/2  "f9o"
